simulink model "EKF"  (R2020b)
settings: Solver=VariableStepAuto  StartTime=0.0  StopTime=20.0  RelTol=1e-3
libraries: simulink x4
settings Model: Creator=ST  LastModifiedBy=DELL

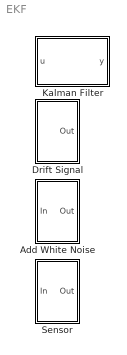
== system EKF ==
  Add White Noise : Subsystem
  Drift Signal : Subsystem
  Kalman Filter : MATLAB Function  TreatAsAtomicUnit=on
  Sensor : Subsystem

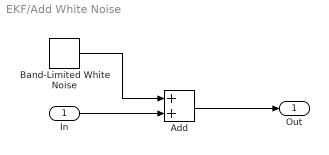
== system EKF/Add White Noise ==
  In : Inport
  Add : Sum
  Band-Limited White Noise : simulink/Sources/Band-Limited White Noise  Cov=[0.1]  Ts=0.1  seed=[23341]
  Out : Outport
  wires:
  Band-Limited White Noise/1 -> Add/1
  In/1 -> Add/2
  Add/1 -> Out/1

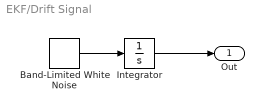
== system EKF/Drift Signal ==
  Band-Limited White Noise : simulink/Sources/Band-Limited White Noise  Cov=[0.1]  Ts=0.1  seed=[23341]
  Integrator : Integrator
  Out : Outport
  wires:
  Band-Limited White Noise/1 -> Integrator/1
  Integrator/1 -> Out/1

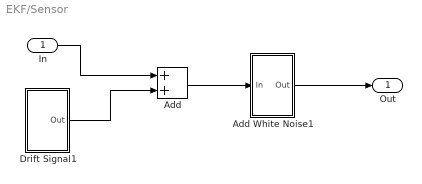
== system EKF/Sensor ==
  In : Inport
  Add : Sum
  Add White Noise1 : Subsystem
  Drift Signal1 : Subsystem
  Out : Outport
  wires:
  Add/1 -> Add White Noise1/1(In)
  Add White Noise1/1(Out) -> Out/1
  Drift Signal1/1(Out) -> Add/2
  In/1 -> Add/1

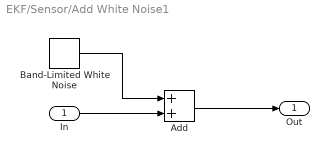
== system EKF/Sensor/Add White Noise1 ==
  In : Inport
  Add : Sum
  Band-Limited White Noise : simulink/Sources/Band-Limited White Noise  Cov=[0.1]  Ts=0.1  seed=[23341]
  Out : Outport
  wires:
  Band-Limited White Noise/1 -> Add/1
  In/1 -> Add/2
  Add/1 -> Out/1

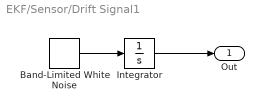
== system EKF/Sensor/Drift Signal1 ==
  Band-Limited White Noise : simulink/Sources/Band-Limited White Noise  Cov=[0.1]  Ts=0.1  seed=[23341]
  Integrator : Integrator
  Out : Outport
  wires:
  Band-Limited White Noise/1 -> Integrator/1
  Integrator/1 -> Out/1

== matlab function EKF/Kalman Filter ==
  data: u input; y output
function y = Kalman_Filter(u)

y = u;
